simulink model "inflowMatrix"  (R2018a)
settings: Solver=ode1  StartTime=0.0  StopTime=1  FixedStep=1/100  RelTol=1e-3
undefined symbols (not defined in the file or in its folder): deg, rad, s
libraries: aerolibconvert2 x6
settings Model: Creator=ali  LastModifiedBy=ali

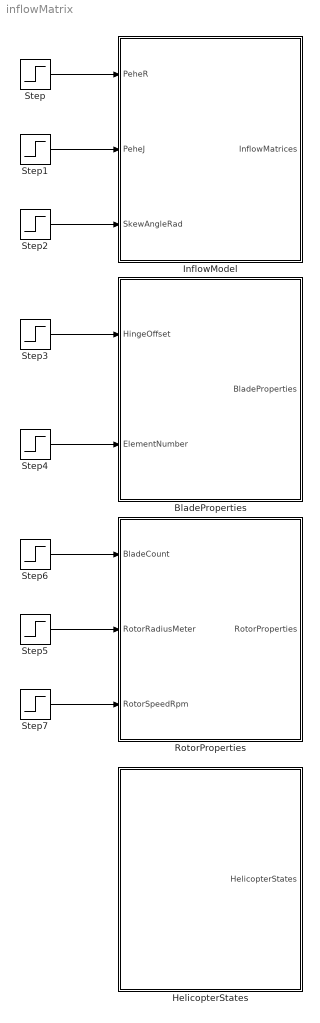
== system inflowMatrix ==
  BladeProperties : Subsystem  TreatAsAtomicUnit=on
  HelicopterStates : Subsystem  TreatAsAtomicUnit=on
  InflowModel : Subsystem  TreatAsAtomicUnit=on
  RotorProperties : Subsystem  TreatAsAtomicUnit=on
  Step : Step  Time=0.5  Before=2  After=4  SampleTime=0
  Step1 : Step  Time=0.5  Before=3  After=2  SampleTime=0
  Step2 : Step  Time=0.5  Before=5.0 * 180.0 / pi  After=-5.0 * 180.0 / pi  SampleTime=0
  Step3 : Step  Time=0.5  Before=0.01  After=0.04  SampleTime=0
  Step4 : Step  Time=0.5  Before=10  After=100  SampleTime=0
  Step5 : Step  Time=0.5  Before=8  After=12  SampleTime=0
  Step6 : Step  Time=0.5  Before=3  After=5  SampleTime=0
  Step7 : Step  Time=0.5  Before=300  After=360  SampleTime=0
  wires:
  Step/1 -> InflowModel/1(PeheR)
  Step1/1 -> InflowModel/2(PeheJ)
  Step2/1 -> InflowModel/3(SkewAngleRad)
  Step3/1 -> BladeProperties/1(HingeOffset)
  Step4/1 -> BladeProperties/2(ElementNumber)
  Step5/1 -> RotorProperties/2(RotorRadiusMeter)
  Step6/1 -> RotorProperties/1(BladeCount)
  Step7/1 -> RotorProperties/3(RotorSpeedRpm)

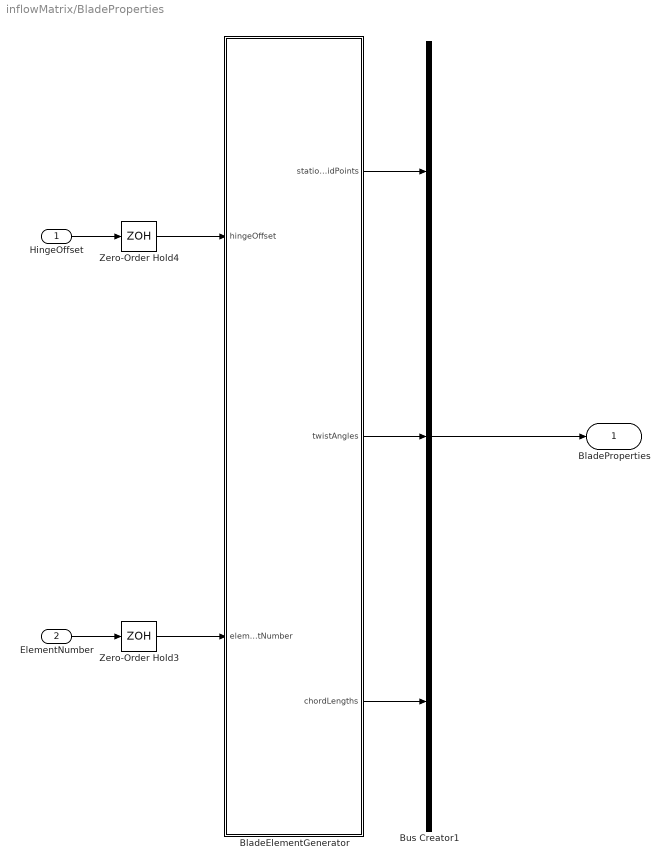
== system inflowMatrix/BladeProperties ==
  HingeOffset : Inport  OutDataTypeStr=double
  ElementNumber : Inport  Port=2  OutDataTypeStr=double
  BladeElementGenerator : MATLAB Function  TreatAsAtomicUnit=on
  Bus Creator1 : BusCreator  Inputs=3
  Zero-Order Hold3 : ZeroOrderHold  SampleTime=-1
  Zero-Order Hold4 : ZeroOrderHold  SampleTime=-1
  BladeProperties : Outport
  wires:
  Zero-Order Hold3/1 -> BladeElementGenerator/2(elementNumber)
  Zero-Order Hold4/1 -> BladeElementGenerator/1(hingeOffset)
  BladeElementGenerator/1(stationMidPoints) -> Bus Creator1/1
  HingeOffset/1 -> Zero-Order Hold4/1
  ElementNumber/1 -> Zero-Order Hold3/1
  BladeElementGenerator/2(twistAngles) -> Bus Creator1/2
  BladeElementGenerator/3(chordLengths) -> Bus Creator1/3
  Bus Creator1/1 -> BladeProperties/1

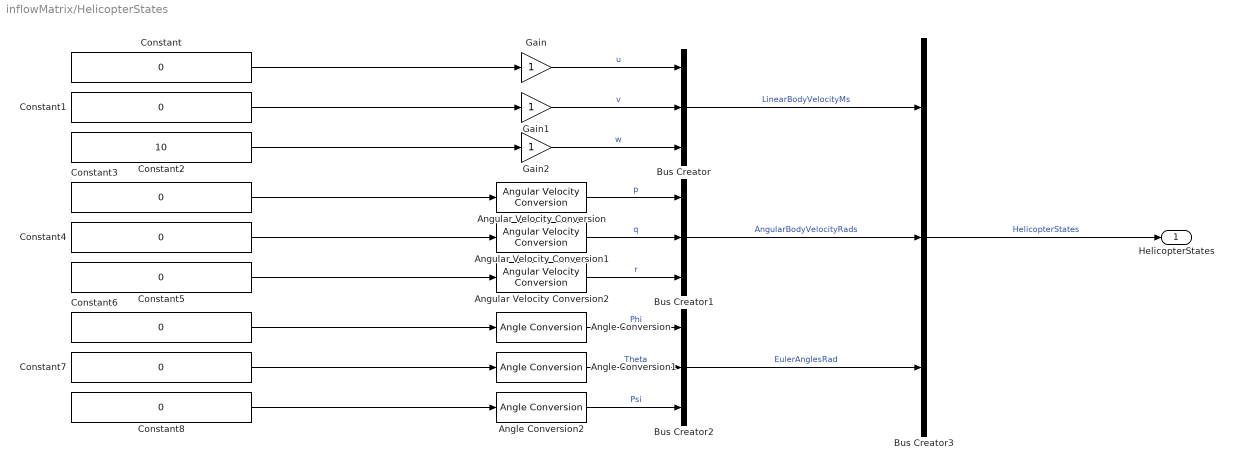
== system inflowMatrix/HelicopterStates ==
  Angle Conversion : aerolibconvert2/Angle Conversion  IU=deg  OU=rad
  Angle Conversion1 : aerolibconvert2/Angle Conversion  IU=deg  OU=rad
  Angle Conversion2 : aerolibconvert2/Angle Conversion  IU=deg  OU=rad
  Angular Velocity Conversion : aerolibconvert2/Angular Velocity Conversion  IU=deg/s  OU=rad/s
      settings: SourceProductName=Aerospace Blockset
  Angular Velocity Conversion1 : aerolibconvert2/Angular Velocity Conversion  IU=deg/s  OU=rad/s
      settings: SourceProductName=Aerospace Blockset
  Angular Velocity Conversion2 : aerolibconvert2/Angular Velocity Conversion  IU=deg/s  OU=rad/s
      settings: SourceProductName=Aerospace Blockset
  Bus Creator{,1..3} (4 alike) : BusCreator  Inputs=3
  Constant{,1,3..8} (8 alike) : Constant  Value=0
  Constant2 : Constant  Value=10
  Gain : Gain
  Gain1 : Gain
  Gain2 : Gain
  HelicopterStates : Outport
  wires:
  Bus Creator/1 -> Bus Creator3/1  "LinearBodyVelocityMs"
  Constant/1 -> Gain/1
  Constant1/1 -> Gain1/1
  Constant2/1 -> Gain2/1
  Gain/1 -> Bus Creator/1  "u"
  Gain1/1 -> Bus Creator/2  "v"
  Gain2/1 -> Bus Creator/3  "w"
  Constant3/1 -> Angular Velocity Conversion/1
  Constant4/1 -> Angular Velocity Conversion1/1
  Constant5/1 -> Angular Velocity Conversion2/1
  Angular Velocity Conversion/1 -> Bus Creator1/1  "p"
  Angular Velocity Conversion1/1 -> Bus Creator1/2  "q"
  Angular Velocity Conversion2/1 -> Bus Creator1/3  "r"
  Constant6/1 -> Angle Conversion/1
  Constant7/1 -> Angle Conversion1/1
  Constant8/1 -> Angle Conversion2/1
  Angle Conversion/1 -> Bus Creator2/1  "Phi"
  Angle Conversion1/1 -> Bus Creator2/2  "Theta"
  Angle Conversion2/1 -> Bus Creator2/3  "Psi"
  Bus Creator1/1 -> Bus Creator3/2  "AngularBodyVelocityRads"
  Bus Creator2/1 -> Bus Creator3/3  "EulerAnglesRad"
  Bus Creator3/1 -> HelicopterStates/1  "HelicopterStates"

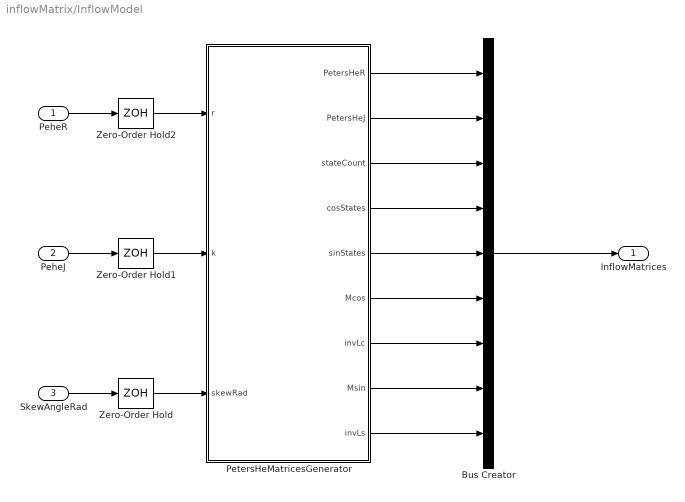
== system inflowMatrix/InflowModel ==
  PeheR : Inport
  PeheJ : Inport  Port=2
  SkewAngleRad : Inport  Port=3
  Bus Creator : BusCreator  Inputs=9
  PetersHeMatricesGenerator : MATLAB Function  TreatAsAtomicUnit=on
  Zero-Order Hold : ZeroOrderHold  SampleTime=-1
  Zero-Order Hold1 : ZeroOrderHold  SampleTime=-1
  Zero-Order Hold2 : ZeroOrderHold  SampleTime=-1
  InflowMatrices : Outport
  wires:
  Zero-Order Hold1/1 -> PetersHeMatricesGenerator/2(k)
  Zero-Order Hold/1 -> PetersHeMatricesGenerator/3(skewRad)
  PeheR/1 -> Zero-Order Hold2/1
  SkewAngleRad/1 -> Zero-Order Hold/1
  Zero-Order Hold2/1 -> PetersHeMatricesGenerator/1(r)
  PeheJ/1 -> Zero-Order Hold1/1
  PetersHeMatricesGenerator/4(cosStates) -> Bus Creator/4
  PetersHeMatricesGenerator/5(sinStates) -> Bus Creator/5
  PetersHeMatricesGenerator/6(Mcos) -> Bus Creator/6
  PetersHeMatricesGenerator/7(invLc) -> Bus Creator/7
  PetersHeMatricesGenerator/8(Msin) -> Bus Creator/8
  PetersHeMatricesGenerator/9(invLs) -> Bus Creator/9
  PetersHeMatricesGenerator/3(stateCount) -> Bus Creator/3
  PetersHeMatricesGenerator/1(PetersHeR) -> Bus Creator/1
  PetersHeMatricesGenerator/2(PetersHeJ) -> Bus Creator/2
  Bus Creator/1 -> InflowMatrices/1

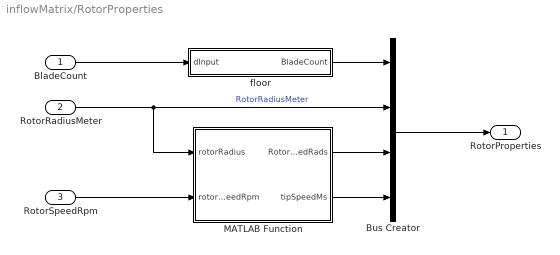
== system inflowMatrix/RotorProperties ==
  BladeCount : Inport  OutDataTypeStr=double
  RotorRadiusMeter : Inport  Port=2  OutDataTypeStr=double
  RotorSpeedRpm : Inport  Port=3  OutDataTypeStr=double
  Bus Creator : BusCreator  Inputs=4
  MATLAB Function : MATLAB Function  TreatAsAtomicUnit=on
  floor : MATLAB Function  TreatAsAtomicUnit=on
  RotorProperties : Outport
  wires:
  RotorSpeedRpm/1 -> MATLAB Function/2(rotorSpeedRpm)
  MATLAB Function/1(RotorSpeedRads) -> Bus Creator/3
  RotorRadiusMeter/1 -> Bus Creator/2, MATLAB Function/1(rotorRadius)  "RotorRadiusMeter"
  MATLAB Function/2(tipSpeedMs) -> Bus Creator/4
  Bus Creator/1 -> RotorProperties/1
  BladeCount/1 -> floor/1(dInput)
  floor/1(BladeCount) -> Bus Creator/1

== matlab function inflowMatrix/BladeProperties/BladeElementGenerator ==
  data: hingeOffset input double; elementNumber input double; stationMidPoints output double size=400; twistAngles output double size=400; chordLengths output double size=400
function [stationMidPoints,twistAngles,chordLengths] = fcn(hingeOffset,elementNumber)

[stationMidPoints]  = readElementNumber(hingeOffset,floor(elementNumber));
[twistAngles]       = readTwist(stationMidPoints);
[chordLengths]      = readChord(stationMidPoints);

== matlab function inflowMatrix/InflowModel/PetersHeMatricesGenerator ==
  data: PetersHeR output double; PetersHeJ output double; stateCount output double; cosStates output double size=60,2; sinStates output double size=60,2; r input double; Mcos output double size=60,60; k input double; skewRad input double; invLc output double size=60,60; Msin output double size=60,60; invLs output double size=60,60
function [PetersHeR,PetersHeJ, stateCount,cosStates,sinStates,Mcos,invLc,Msin,invLs] = fcn(r,k,skewRad)
 PetersHeR = floor(r);
 PetersHeJ = floor(k);
[stateCount,cosStates,sinStates,Mcos,invLc,Msin,invLs] = CreateInflowMatrices(PetersHeR,PetersHeJ,skewRad);

== matlab function inflowMatrix/RotorProperties/MATLAB Function ==
  data: rotorRadius input; RotorSpeedRads output; rotorSpeedRpm input; tipSpeedMs output
function [RotorSpeedRads, tipSpeedMs] = fcn(rotorRadius, rotorSpeedRpm)

RotorSpeedRads = (rotorSpeedRpm / 60.0) * 2.0 * pi;
tipSpeedMs = RotorSpeedRads * rotorRadius;

== matlab function inflowMatrix/RotorProperties/floor ==
  data: dInput input; BladeCount output
function BladeCount  = fcn(dInput)
BladeCount = floor(dInput);
